simulink model "M_v4_GUI"  (R2024b)
settings: Solver=FixedStepAuto  StartTime=0.0  StopTime=solvertime  FixedStep=stepsize  RelTol=1e-3
undefined symbols (not defined in the file or in its folder): pulse_amp, pulse_rate
libraries: Libs_unified x1
settings Model: Creator=ball907  LastModifiedBy=ball907

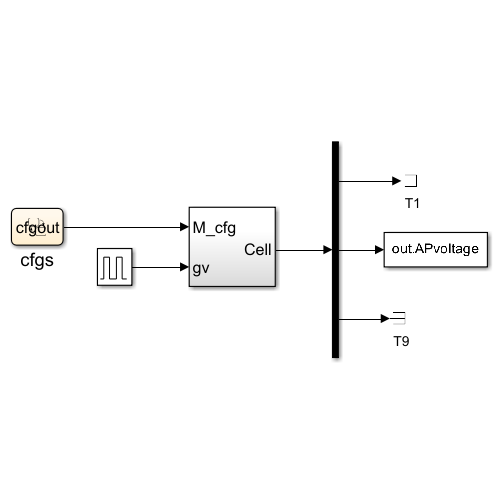
[thumbnail: Simulink's stored preview of the top-level diagram]
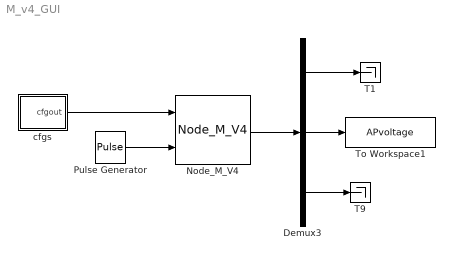
== system M_v4_GUI ==
  Demux3 : Demux  Outputs=[1, 1, 3]
  Node_M_V4 : Libs_unified/Node_M_V4  SystemSampleTime=-1  VariantActivationTime=update diagram  AllowFlexibleInterface=on  Latency=0  AutoFrameSizeCalculation=off
  Pulse Generator : DiscretePulseGenerator  PulseType=Time based  Amplitude=pulse_amp  Period=pulse_rate
  T1 : Terminator
  T9 : Terminator
  To Workspace1 : ToWorkspace  VariableName=APvoltage  SaveFormat=Timeseries  SampleTime=-1
  cfgs : Stateflow chart  TreatAsAtomicUnit=on
  wires:
  Demux3/3 -> T9/1
  Demux3/1 -> T1/1
  Demux3/2 -> To Workspace1/1
  Pulse Generator/1 -> Node_M_V4/2
  cfgs/1(cfgout) -> Node_M_V4/1
  Node_M_V4/1 -> Demux3/1

== stateflow chart M_v4_GUI/cfgs ==
  settings: executeAtInitialization=1
  state Ini
  (default) -> Ini : {cfgout=auto;}
  data: cfg function_output; params parameter; cfgout output
  function cfg = auto:
    | function cfg = auto
    | 
    | ax0=params(1,1);
    | ay0=params(1,2);
    | az0=params(1,3);
    |  
    | ax1=params(1,4);
    | ay1=params(1,5);
    | az1=params(1,6);
    |  
    | ax2=params(1,7);
    | ay2=params(1,8);
    | az2=params(1,9);
    |  
    | ax3=params(1,10);
    | ay3=params(1,11);
    | az3=params(1,12);
    |  
    | bx1=params(1,13);
    | by1=params(1,14);
    | bz1=params(1,15);
    | 
    | VR=params(1,16);
    | VT=params(1,17);
    | VO=params(1,18);
    |  
    | a=params(1,19);
    | b=params(1,20);
    | c=params(1,21);
    | d=params(1,22);
    | e=params(1,23);
    | 
    | x=params(1,23);
    | y=params(1,24);
    | 
    | cfg=[ax0,ay0,az0,ax1,ay1,az1,ax2,ay2,az2,ax3,ay3,az3,bx1,by1,bz1,VR,VT,VO,a,b,c,d,e,x,y];
    | end
